simulink library "MPC_51_v1_GP_CL"  (R2018b)
settings: Solver=VariableStepAuto  StartTime=0.0  StopTime=10.0  RelTol=1e-3
libraries: Post_MPC_UL x1, solver_51_v1_UL x1
settings Model: Creator=John Jr  LastModifiedBy=John Jr

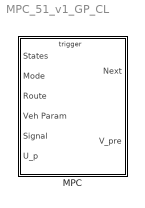
== system MPC_51_v1_GP_CL ==
  MPC : Subsystem  TreatAsAtomicUnit=on
      mask Display:
      | patch([0 1 1 0], [0 0 1 1],[1 .8 1])
      | 
      | port_label('input',1,'\fontname{Cambria Math}States','texmode','on')
      | port_label('input',2,'\fontname{Cambria Math}Mode','texmode','on')
      | port_label('input',3,'\fontname{Cambria Math}Route','texmode','on')
      | port_label('input',4,'\fontname{Cambria Math}Param','texmode','on')
      | port_label('input',5,'\fontname{Cambria Math}Signal','texmode','on')
      | port_label('input',6,'\fontname{Cambria Math}U_{pre}','texmode','on')
      | 
      | port_label('output',1,'\fontname{Cambria Math}V_{MPC},T_{MPC}','texmode','on')
      | port_label('output',2,'\fontname{Cambria Math}V_{pre}','texmode','on')
      | 
      | port_label('trigger','\spadesuit','texmode','on')
      | 
      | disp('\fontname{Cambria Math}\fontsize{12}  MPC v1\newline  51 Step','texmode','on')

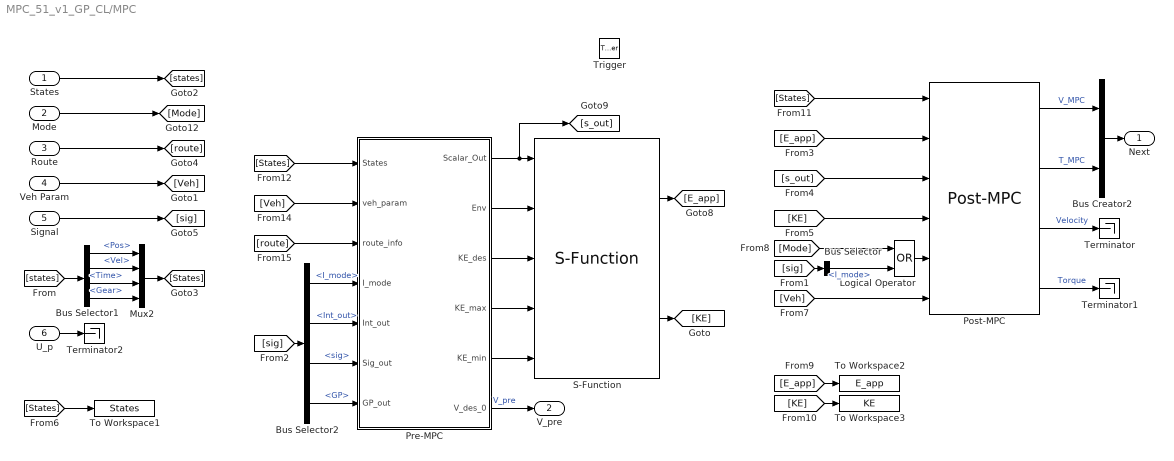
== system MPC_51_v1_GP_CL/MPC ==
  States : Inport
  Mode : Inport  Port=2
  Route : Inport  Port=3
  Veh Param : Inport  Port=4
  Signal : Inport  Port=5
  U_p : Inport  Port=6
  Trigger : TriggerPort  TriggerType=falling  VariantControl=Variant
  Bus Creator2 : BusCreator  Inputs=2
  Bus Selector : BusSelector  OutputSignals=Signal.I_mode
  Bus Selector1 : BusSelector  OutputSignals=Pos,Vel,Time,Gear
  Bus Selector2 : BusSelector  OutputSignals=Signal.I_mode,Signal.Int_out,Signal.sig,GP
  Logical Operator : Logic  Operator=OR  AllPortsSameDT=off  OutDataTypeStr=boolean
  Mux2 : Mux
  Post-MPC : Post_MPC_UL/Post-MPC  SystemSampleTime=-1
  Pre-MPC : MATLAB Function  TreatAsAtomicUnit=on
  S-Function : solver_51_v1_UL/S-Function  SFunctionModules=solver_51_v1_wrapper
  Terminator : Terminator
  Terminator1 : Terminator
  Terminator2 : Terminator
  To Workspace1 : ToWorkspace  VariableName=States  SampleTime=-1
  To Workspace2 : ToWorkspace  VariableName=E_app  SampleTime=-1
  To Workspace3 : ToWorkspace  VariableName=KE  SampleTime=-1
  Next : Outport
  V_pre : Outport  Port=2
  wires:
  Bus Selector2/1 -> Pre-MPC/4(I_mode)  "<I_mode>"
  Bus Selector2/2 -> Pre-MPC/5(Int_out)  "<Int_out>"
  Bus Selector2/3 -> Pre-MPC/6(Sig_out)  "<sig>"
  Bus Selector2/4 -> Pre-MPC/7(GP_out)  "<GP>"
  [sig] -> Bus Selector2/1
  Pre-MPC/6(V_des_0) -> V_pre/1  "V_pre"
  Bus Selector/1 -> Logical Operator/2  "<I_mode>"
  [sig] -> Bus Selector/1
  [Mode] -> Logical Operator/1
  States/1 -> [states]
  Route/1 -> [route]
  Bus Selector1/4 -> Mux2/4  "<Gear>"
  Bus Selector1/2 -> Mux2/2  "<Vel>"
  Bus Selector1/3 -> Mux2/3  "<Time>"
  Bus Selector1/1 -> Mux2/1  "<Pos>"
  [states] -> Bus Selector1/1
  Veh Param/1 -> [Veh]
  [Veh] -> Post-MPC/6
  Post-MPC/4 -> Terminator1/1  "Torque"
  Post-MPC/3 -> Terminator/1  "Velocity"
  Mux2/1 -> [States]
  [States] -> Pre-MPC/1(States)
  [States] -> Post-MPC/1
  [Veh] -> Pre-MPC/2(veh_param)
  [route] -> Pre-MPC/3(route_info)
  Mode/1 -> [Mode]
  Pre-MPC/4(KE_max) -> S-Function/4
  Pre-MPC/5(KE_min) -> S-Function/5
  [E_app] -> Post-MPC/2
  [s_out] -> Post-MPC/3
  [KE] -> Post-MPC/4
  Pre-MPC/1(Scalar_Out) -> S-Function/1, [s_out]
  Logical Operator/1 -> Post-MPC/5
  S-Function/2 -> [KE]
  S-Function/1 -> [E_app]
  Pre-MPC/2(Env) -> S-Function/2
  Pre-MPC/3(KE_des) -> S-Function/3
  [States] -> To Workspace1/1
  Bus Creator2/1 -> Next/1
  Post-MPC/1 -> Bus Creator2/1  "V_MPC"
  Post-MPC/2 -> Bus Creator2/2  "T_MPC"
  Signal/1 -> [sig]
  U_p/1 -> Terminator2/1
  [E_app] -> To Workspace2/1
  [KE] -> To Workspace3/1

== matlab function MPC_51_v1_GP_CL/MPC/Pre-MPC ==
  data: States input size=4; Scalar_Out output; Env output; veh_param input; route_info input; I_mode input; Int_out input; KE_des output; KE_max output; KE_min output; V_des_0 output; Sig_out input; GP_out input
function [Scalar_Out,Env,KE_des,KE_max,KE_min,V_des_0] = ...
    fcn(States,veh_param,route_info,I_mode,Int_out,Sig_out,GP_out)

t_0 = States(3);                                        %   s - Sim time
if t_0 == 0
    t_0 = .01;
end
x_0 = States(1);                                        %   m - Current position
v_0 = States(2);                                        %   m/s - Current velocity 
GR = States(4);                                         %   Current Gear
g = veh_param(1);                                       %   m/s^2 - Accel due to gravity
rho = veh_param(2);                                     %   kg/m^3 - Air density
m = veh_param(3);                                       %   kg - Base vehicle mass
Cd = veh_param(4);                                      %   Drag Coefficient
A_ref = veh_param(5);                                   %   m^2 - Reference area
Cr = veh_param(6);                                      %   Rolling resistance coefficient
r_wh = veh_param(7);                                    %   m - Wheel radius
X_vec = route_info(:,1);                                %   rad - Road grade angle vector
theta_vec = route_info(:,2);                            %   rad - Road grade angle vector
V_lim = route_info(:,3);                                %   m/s - Current speed limit
v_DP = route_info(:,4);                                 %   m/s - Offline optimized velocity                                       


%%  Controller Setup
dx = 10;                                                %   m - Position step
N = 51;                                                 %   # of pred steps
x_pred = dx*N;                                          %   m - Prediction horizon length
xp_vec = (x_0:dx:x_0+x_pred)';                          %   m - Position vector

%%  Horizon Vectors
V_des = zeros(N,1);                                     %   m/s - Initialize des velocty vector
V_des_0 = 0;                                            %   m/s - Initialize 1st desired velocity
v_lim = interp1(X_vec,V_lim,xp_vec(1:N),...             %   m/s - Maximum velocity vector 
    'linear',V_lim(end));
v_min = 0*v_lim;                                        %   m/s - Minimum velocity vector 
theta = interp1(X_vec,theta_vec,xp_vec(1:N),...         %   rad - Road grade vector 
    'linear',theta_vec(end));
KE_max = .5*m*v_lim.^2;                                 %   J - Maximum kinetic energy vector 
KE_min = .5*m*v_min.^2;                                 %   J - Minimum kinetic energy vector 
F_grav = m*g*sin(theta);                                %   N - Gravitational force vector 
F_road = m*g*Cr*cos(theta);                             %   N - Rolling resistance force vector 
Env = (F_road+F_grav)*dx;                               %   J - Environmental resistance energy vector 

%%  Intersection properties
if I_mode == 1
    [G_in,R_in,Cs_p,Cs_V] = getGRvec(Int_out,Sig_out,GP_out);
    NI = length(Int_out(isnan(Int_out(:,1))==0));       %   # of upcoming intersections
    M = length(G_in(1,:));                              %   # of green and red times
    pG = zeros(NI,M);
    tG = zeros(NI,M);
    Int_dx = zeros(NI,1);                               %   m - Initialize distance to intersections vector 
    Int_ds = zeros(NI,1);                               %   m - Initialize distance between intersections vector 
    G = zeros(NI,M);                                    %   m - Initialize green time vector 
    R = zeros(NI,M);                                    %   m - Initialize red time vector 
    for i = 1:NI
        [t_ref,pGreen] = getProb(i,Sig_out,Int_out,GP_out,Cs_p,Cs_V);
        [pG(i,:),tG(i,:)] = findpeaks(pGreen,t_ref);
        Int_dx(i) = Int_out(i,2);                       %   m - Distance to intersections
        Int_ds(i) = Int_out(i,3);                       %   m - Distance between intersections
        G(i,:) = G_in(i,:);                             %   s - Time light turns green
        R(i,:) = R_in(i,:);                             %   s - Time light turns red
    end
    Int_x = x_0+Int_dx;                                 %   m - Intersection locations
    C_cur = zeros(NI,1);
    Red_Light = zeros(NI,1);                            %   Initialize red light vector
    v_max_adj = zeros(NI,1);                            %   m/s - Initialize max vel adj vector
    v_min_adj = zeros(NI,1);                            %   m/s - Initialize min vel adj vector
    v_des = zeros(NI,1);                                %   m/s - Initialize desired velocity vector
    G_dt = zeros(NI,M);                                 %   s - Time to green
    G_dt1 = zeros(NI,M);                                %   s - Time to green
    v_max_G = zeros(NI,M);                              %   m/s - Velocity to reach light at green 
    v_max_G1 = zeros(NI,M);                             %   m/s - Velocity to reach light at green 
    R_dt = zeros(NI,M);                                 %   s - Time to red
    v_min_R = zeros(NI,M);                              %   m/s - Velocity to reach light at red 
    Int_v_max = interp1(X_vec,V_lim,...                 %   m/s - Intersection max velocity
        Int_x,'linear',V_lim(end));
    Int_v_min = Int_v_max*.25;                          %   m/s - Intersection min velocity
    Int_t = t_0*ones(NI+1,1);                           %   s - Temp time vector for des vel
    Int_t_max = t_0*ones(NI+1,1);                       %   s - Temp time vector for max vel
    Int_t_min = t_0*ones(NI+1,1);                       %   s - Temp time vector for min vel
    for i = 1:NI
        C_cur(i) = find(Int_t(i) > G(i,:),1,'last');    %   s - Current light period
        if Int_t(i) < R(i,C_cur(i))                     %   Check current light status
            Red_Light(i) = 0;                           %   Light is green
        else
            Red_Light(i) = 1;                           %   Light is red
        end
        Int_condition = 0;                              %   Initialize condition
        j = 0;                                          %   Initialize counter
        while Int_condition == 0
            j = j+1;
            if j == M+1
                Int_v_min(i) = max(Int_v_min(i)-1,0);
                j = 1;
            end
            G_dt(i,j) = G(i,j)-Int_t(i);                %   s - Time till light turns green
            v_max_G(i,j) = Int_ds(i)/G_dt(i,j);         %   m/s - Velocity to reach li ght turning green
            G_dt1(i,j) = tG(i,j)-Int_t(i);              %   s - Time till light turns green
            v_max_G1(i,j) = Int_ds(i)/G_dt1(i,j);       %   m/s - Velocity to reach li ght turning green
            R_dt(i,j) = R(i,j)-Int_t(i);                %   s - Time till light turns red
            v_min_R(i,j) = Int_ds(i)/R_dt(i,j);         %   m/s - Velocity to reach light turning red
            if Red_Light(i) == 0 && j == 1 ...
                    && v_max_G1(i,j) < Int_v_max(i)...
                    && v_max_G1(i,j) > 0
                Int_condition = 1;
                v_max_adj(i) = Int_v_max(i);            %   m/s - Adjusted maximum velocity
                v_min_adj(i) = max(v_max_G1(i,j)...      %   m/s - Adjusted minimum velocity
                    ,Int_v_min(i));
                v_des(i) = Int_v_max(i);                %   m/s - Desired velocity 
            elseif v_max_G1(i,j) > Int_v_min(i)...
                    && v_max_G1(i,j) < Int_v_max(i)
                Int_condition = 2;
                v_max_adj(i) = min(Int_v_max(i)...      %   m/s - Adjusted minimum velocity
                    ,v_max_G1(i,j));
                v_min_adj(i) = v_max_G1(i,j);            %   m/s - Adjusted minimum velocity
                v_des(i) = (v_max_adj(i)...             %   m/s - Desired velocity 
                    +v_min_adj(i))/2;
            elseif v_max_G1(i,j) < Int_v_max(i)...
                    && v_max_G1(i,j) > Int_v_min(i)
                Int_condition = 4;
                v_max_adj(i) = v_max_G1(i,j);            %   m/s - Adjusted minimum velocity
                v_min_adj(i) = max(Int_v_min(i),...     %   m/s - Adjusted minimum velocity
                    v_max_G1(i,j));        
                v_des(i) = v_max_G1(i,j);                %   m/s - Desired velocity 
            end
        end
        Int_t(i+1) = Int_ds(i)/v_des(i)+Int_t(i);       %   s - Desired velocity time vector
        Int_t_max(i+1) = Int_ds(i)/v_max_adj(i)...      %   s - Max velocity time vector
            +Int_t_max(i);
        Int_t_min(i+1) = Int_ds(i)/v_min_adj(i)...      %   s - Min velocity time vector
            +Int_t_min(i); 
    end
    for i = 1:N
        V_des(i) = interp1([x_0;Int_x],...              %   m/s - Desired velocity through intersections 
            [v_des;v_des(end)],xp_vec(i),...
            'previous','extrap');
        V_des_0 = V_des(1);
    end
else
    Int_x = NaN;
    for i = 1:N
        V_des(i) = interp1(X_vec,v_DP,xp_vec(i),...
            'linear',v_DP(end));
        V_des_0 = V_des(1);
    end
end

A = 1-1/m*rho*Cd*A_ref*dx;                              %   Dynamics matrix
KE_0 = 1/2*m*v_0^2;                                     %   J - Initial kinetic energy 
F_wh_max = min(2200.*2.47*GR/r_wh,80000);               %   N - Maximum control force
E_mech_max = F_wh_max*dx;                               %   J - Initial max ME
E_mech_min = 0;                                         %   J - Mechanical energy lower limit 
E_brk_max = 35000*dx;                                   %   J - Brake energy upper limit 
E_brk_min = 0;                                          %   J - Brake energy lower limit 
KE_des = 1/2*m.*V_des.^2;                               %   J - Initialize desired KE vector
lam_e = zeros(N,1); lam_b = zeros(N,1);
[lam_e(:,1),lam_b(:,1)] = getWeights(xp_vec,Int_x,I_mode);        %   Objective weights

Scalar_Out = [A,KE_0,E_mech_max,E_mech_min,...
    E_brk_max,E_brk_min,lam_e(1),lam_b(1)]';
